simulink model "model2"  (R2024a)
settings: Solver=VariableStepAuto  StartTime=0.0  StopTime=10.0  RelTol=1e-3
values from neighbouring files (symbols this model uses):
  A = 1    [modelSaxe.m]    (also in script1.m = [-40  16   9   7; script2.m = [-40  16   9   7; script3.m = [-40  16   9   7)
  C = 1    [modelSaxe.m]    (also in script1.m = [-3  2  -2  1]; script2.m = [-3  2  -2  1]; script3.m = [-3  2  -2  1])
  L = 1    [modelSaxe.m]    (also in script1.m = T^-1 * L_k; script2.m = T^-1 * L_k; script3.m = T^-1 * L_k)
settings Model: Creator=eva  LastModifiedBy=eva

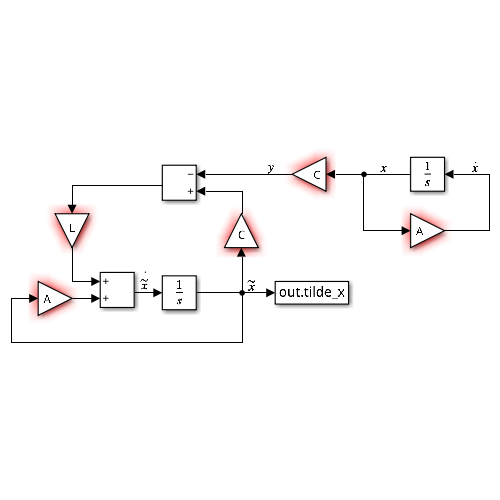
[thumbnail: Simulink's stored preview of the top-level diagram]
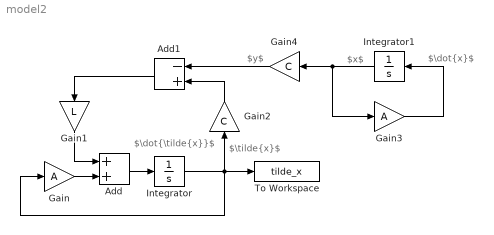
== system model2 ==
  note: $\dot{x}$
  note: $x$
  note: $y$
  note: $\tilde{x}$
  note: $\dot{\tilde{x}}$
  Add : Sum
  Add1 : Sum  Inputs=-+
  Gain : Gain  Gain=A
  Gain1 : Gain  Gain=L
  Gain2 : Gain  Gain=C
  Gain3 : Gain  Gain=A
  Gain4 : Gain  Gain=C
  Integrator : Integrator
  Integrator1 : Integrator
  To Workspace : ToWorkspace  VariableName=tilde_x  SaveFormat=Timeseries  SampleTime=-1
  wires:
  Integrator/1 -> Gain2/1, To Workspace/1, Gain/1
  Add/1 -> Integrator/1
  Gain/1 -> Add/2
  Gain1/1 -> Add/1
  Gain2/1 -> Add1/2
  Add1/1 -> Gain1/1
  Integrator1/1 -> Gain4/1, Gain3/1
  Gain3/1 -> Integrator1/1
  Gain4/1 -> Add1/1
